simulink model "sampleModel1409"  (R2023a)
settings: Solver=VariableStepAuto  StartTime=0.0  StopTime=10.0  RelTol=1e-3
libraries: hdlsllib x3, simulink x1
settings Model: Creator=user1  LastModifiedBy=user1

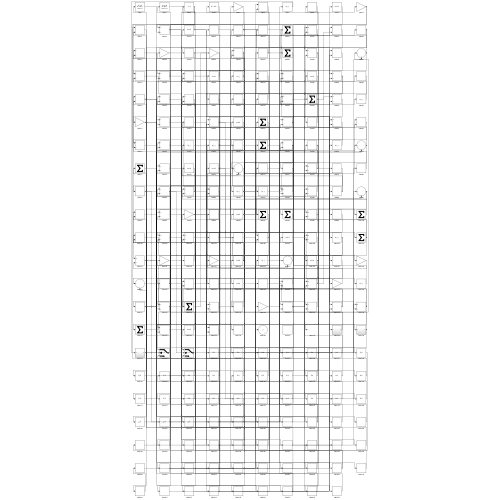
[thumbnail: Simulink's stored preview of the top-level diagram]
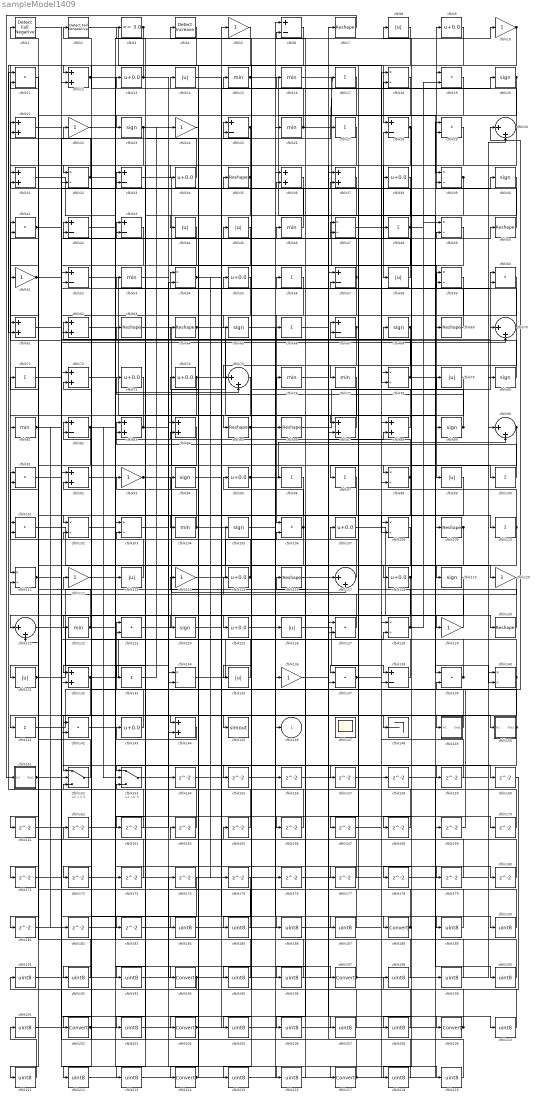
== system sampleModel1409 ==
  cfblk1 : hdlsllib/Logic and Bit Operations/Detect Fall Negative  vinit=0  OutDataTypeStr=boolean
  cfblk{5,10,22,24,51,93,112,114,120,129,136} (11 alike) : Gain
  cfblk{17,27,48,56,66,71,96..97,100,110,133,141} (12 alike) : Sum  Inputs=+
  cfblk{11,19,29,41,60,91,101,106,123,127,137,139,142} (13 alike) : DotProduct  OutDataTypeStr=Inherit: Inherit via internal rule
  cfblk{18,32,39,47,49,54,59,78,98,102..103,108,111,128,134,140} (16 alike) : Product  Inputs=*/  RndMeth=Zero  SaturateOnIntegerOverflow=on
  cfblk{15..16,26,46,53,76..77,81,104,122} (10 alike) : MinMax
  cfblk{20,23,40,65,68,80,89,94,105,119,124} (11 alike) : Signum
  cfblk{9,13,34,38,55,73..74,95,107,115,118,125,143} (13 alike) : Bias  Bias=0.0  SaturateOnIntegerOverflow=off
  cfblk{7,35,50,63..64,69,85..86,109,116,130} (11 alike) : Reshape
  cfblk{8,14,44..45,58,79,99,113,126,131,135} (11 alike) : Abs  SaturateOnIntegerOverflow=off
  cfblk{30,70,75,90,117,121} (6 alike) : Sum  Inputs=|++
  cfblk{12,21,31,36..37,61..62,72,83..84,87..88,92,132,144} (15 alike) : Sum
  cfblk{6,25,28,33,42..43,52,57,67,82,138} (11 alike) : Sum  Inputs=+-
  cfblk145 : ToWorkspace  VariableName=simout  SaveFormat=Timeseries  SampleTime=-1
  cfblk147 : Scope
      settings: Floating=on
  cfblk148 : Terminator
  cfblk149 : Subsystem
      settings: LibrarySourceBlock=|
      | hdlsllib/Ports &
      | Subsystems/Subsystem
  cfblk150 : Subsystem
      settings: LibrarySourceBlock=|
      | hdlsllib/Ports &
      | Subsystems/Subsystem
  cfblk151 : Subsystem
      settings: LibrarySourceBlock=|
      | hdlsllib/Ports &
      | Subsystems/Subsystem
  cfblk152 : Switch  SaturateOnIntegerOverflow=off  InputSameDT=off
  cfblk153 : Switch  SaturateOnIntegerOverflow=off  InputSameDT=off
  cfblk{154..183} (30 alike) : Delay  SampleTime=1
  cfblk{184..187,189..193,195..196,198..201,203,205..208,210..213,215..216,218..219} (28 alike) : DataTypeConversion  OutDataTypeStr=uint8  SaturateOnIntegerOverflow=off  RndMeth=Floor
  cfblk{188,194,197,202,204,209,214,217} (8 alike) : DataTypeConversion  SaturateOnIntegerOverflow=off  RndMeth=Floor
  cfblk2 : hdlsllib/Logic and Bit Operations/Detect Fall Nonpositive  vinit=0  OutDataTypeStr=boolean
  cfblk3 : hdlsllib/Logic and Bit Operations/Compare To Constant  relop=<=  const=3.0  OutDataTypeStr=boolean
  cfblk4 : simulink/Logic and Bit Operations/Detect Increase  vinit=0.0  OutDataTypeStr=boolean
      settings: LibrarySourceBlock=|
      | hdlsllib/Logic and Bit
      | Operations/Detect
      | Increase
  cfblk146 : Outport  VectorParamsAs1DForOutWhenUnconnected=off
  wires:
  cfblk4/1 -> cfblk111/1
  cfblk133/1 -> cfblk24/1
  cfblk90/1 -> cfblk83/2, cfblk208/1
  cfblk28/1 -> cfblk87/2, cfblk168/1
  cfblk63/1 -> cfblk98/1
  cfblk51/1 -> cfblk160/1, cfblk161/1, cfblk187/1
  cfblk141/1 -> cfblk30/1
  cfblk35/1 -> cfblk34/1, cfblk183/1
  cfblk52/1 -> cfblk85/1
  cfblk30/1 -> cfblk15/1, cfblk58/1
  cfblk83/1 -> cfblk81/1, cfblk100/1
  cfblk93/1 -> cfblk117/2, cfblk43/2, cfblk67/1
  cfblk128/1 -> cfblk62/1, cfblk19/2
  cfblk67/1 -> cfblk125/1, cfblk215/1
  cfblk16/1 -> cfblk99/1
  cfblk135/1 -> cfblk83/1
  cfblk126/1 -> cfblk138/1
  cfblk64/1 -> cfblk109/1, cfblk96/1
  cfblk14/1 -> cfblk188/1
  cfblk7/1 -> cfblk151/1(In1)
  cfblk104/1 -> cfblk33/1, cfblk120/1
  cfblk140/1 -> cfblk152/1, cfblk56/1, cfblk114/1
  cfblk113/1 -> cfblk91/1
  cfblk99/1 -> cfblk144/1
  cfblk59/1 -> cfblk106/1
  cfblk107/1 -> cfblk130/1
  cfblk132/1 -> cfblk108/1, cfblk171/1
  cfblk70/1 -> cfblk18/2, cfblk157/1
  cfblk32/1 -> cfblk21/1, cfblk108/2
  cfblk121/1 -> cfblk134/2
  cfblk10/1 -> cfblk77/1, cfblk61/2
  cfblk144/1 -> cfblk143/1
  cfblk82/1 -> cfblk121/1, cfblk153/2, cfblk49/2
  cfblk103/1 -> cfblk197/1
  cfblk120/1 -> cfblk111/2
  cfblk88/1 -> cfblk54/1
  cfblk152/1 -> cfblk71/1
  cfblk87/1 -> cfblk4/1
  cfblk109/1 -> cfblk148/1, cfblk131/1
  cfblk11/1 -> cfblk31/1
  cfblk150/1(Out1) -> cfblk42/1, cfblk193/1
  cfblk6/1 -> cfblk204/1
  cfblk36/1 -> cfblk214/1
  cfblk89/1 -> cfblk64/1, cfblk73/1
  cfblk114/1 -> cfblk106/2
  cfblk101/1 -> cfblk119/1
  cfblk58/1 -> cfblk42/2
  cfblk95/1 -> cfblk90/2, cfblk38/1
  cfblk84/1 -> cfblk152/2
  cfblk33/1 -> cfblk89/1
  cfblk26/1 -> cfblk17/1, cfblk2/1
  cfblk50/1 -> cfblk9/1
  cfblk74/1 -> cfblk136/1, cfblk142/2, cfblk175/1
  cfblk124/1 -> cfblk20/1
  cfblk18/1 -> cfblk23/1
  cfblk149/1(Out1) -> cfblk25/1
  cfblk48/1 -> cfblk13/1, cfblk102/1, cfblk49/1
  cfblk46/1 -> cfblk31/2
  cfblk80/1 -> cfblk41/1
  cfblk12/1 -> cfblk145/1, cfblk110/1
  cfblk119/1 -> cfblk141/1
  cfblk55/1 -> cfblk65/1
  cfblk138/1 -> cfblk95/1
  cfblk40/1 -> cfblk97/1
  cfblk27/1 -> cfblk61/1
  cfblk106/1 -> cfblk45/1, cfblk213/1
  cfblk131/1 -> cfblk88/2, cfblk48/1, cfblk70/2
  cfblk123/1 -> cfblk68/1
  cfblk21/1 -> cfblk129/1
  cfblk117/1 -> cfblk107/1
  cfblk75/1 -> cfblk122/1
  cfblk86/1 -> cfblk60/1
  cfblk73/1 -> cfblk142/1
  cfblk92/1 -> cfblk217/1
  cfblk98/1 -> cfblk53/1, cfblk206/1
  cfblk111/1 -> cfblk55/1, cfblk70/1
  cfblk23/1 -> cfblk212/1, cfblk216/1
  cfblk143/1 -> cfblk123/1
  cfblk56/1 -> cfblk144/2
  cfblk136/1 -> cfblk7/1
  cfblk68/1 -> cfblk135/1, cfblk178/1
  cfblk142/1 -> cfblk60/2
  cfblk76/1 -> cfblk209/1
  cfblk39/1 -> cfblk137/1, cfblk44/1
  cfblk45/1 -> cfblk124/1
  cfblk31/1 -> cfblk113/1
  cfblk72/1 -> cfblk194/1
  cfblk25/1 -> cfblk132/1, cfblk133/1
  cfblk85/1 -> cfblk57/2, cfblk170/1
  cfblk24/1 -> cfblk104/1
  cfblk139/1 -> cfblk82/1, cfblk16/1
  cfblk9/1 -> cfblk28/1
  cfblk110/1 -> cfblk118/1, cfblk67/2, cfblk47/2
  cfblk61/1 -> cfblk40/1
  cfblk47/1 -> cfblk28/2
  cfblk79/1 -> cfblk86/1
  cfblk115/1 -> cfblk63/1, cfblk102/2
  cfblk2/1 -> cfblk78/2
  cfblk153/1 -> cfblk69/1
  cfblk137/1 -> cfblk79/1, cfblk50/1
  cfblk122/1 -> cfblk11/2, cfblk166/1
  cfblk94/1 -> cfblk59/1
  cfblk62/1 -> cfblk10/1
  cfblk118/1 -> cfblk8/1, cfblk137/2
  cfblk100/1 -> cfblk35/1
  cfblk41/1 -> cfblk52/1, cfblk150/1(In1)
  cfblk97/1 -> cfblk153/1
  cfblk8/1 -> cfblk75/1
  cfblk78/1 -> cfblk46/1, cfblk140/2
  cfblk22/1 -> cfblk75/2
  cfblk69/1 -> cfblk43/1
  cfblk81/1 -> cfblk149/1(In1), cfblk182/1
  cfblk13/1 -> cfblk59/2, cfblk12/1, cfblk180/1
  cfblk116/1 -> cfblk19/1
  cfblk151/1(Out1) -> cfblk128/2, cfblk27/1
  cfblk19/1 -> cfblk51/1
  cfblk57/1 -> cfblk132/2, cfblk47/1
  cfblk127/1 -> cfblk84/2
  cfblk15/1 -> cfblk139/1, cfblk39/1
  cfblk3/1 -> cfblk32/1, cfblk12/2
  cfblk43/1 -> cfblk52/2
  cfblk134/1 -> cfblk26/1
  cfblk17/1 -> cfblk32/2
  cfblk34/1 -> cfblk3/1
  cfblk130/1 -> cfblk101/1
  cfblk20/1 -> cfblk87/1, cfblk155/1
  cfblk54/1 -> cfblk105/1, cfblk159/1
  cfblk5/1 -> cfblk202/1
  cfblk129/1 -> cfblk115/1
  cfblk53/1 -> cfblk154/1
  cfblk154/1 -> cfblk90/1
  cfblk155/1 -> cfblk138/2
  cfblk65/1 -> cfblk156/1
  cfblk157/1 -> cfblk30/2
  cfblk159/1 -> cfblk18/1
  cfblk161/1 -> cfblk54/2
  cfblk37/1 -> cfblk163/1
  cfblk163/1 -> cfblk11/1
  cfblk164/1 -> cfblk91/2
  cfblk165/1 -> cfblk121/2
  cfblk166/1 -> cfblk152/3
  cfblk60/1 -> cfblk167/1
  cfblk167/1 -> cfblk128/1
  cfblk168/1 -> cfblk134/1
  cfblk169/1 -> cfblk139/2
  cfblk170/1 -> cfblk84/1
  cfblk171/1 -> cfblk62/2
  cfblk108/1 -> cfblk172/1
  cfblk172/1 -> cfblk57/1
  cfblk42/1 -> cfblk173/1
  cfblk173/1 -> cfblk82/2
  cfblk176/1 -> cfblk98/2
  cfblk102/1 -> cfblk177/1
  cfblk177/1 -> cfblk21/2
  cfblk178/1 -> cfblk140/1
  cfblk125/1 -> cfblk179/1
  cfblk179/1 -> cfblk33/2
  cfblk180/1 -> cfblk25/2
  cfblk96/1 -> cfblk181/1
  cfblk181/1 -> cfblk78/1
  cfblk182/1 -> cfblk123/2
  cfblk183/1 -> cfblk117/1
  cfblk1/1 -> cfblk184/1
  cfblk184/1 -> cfblk126/1
  cfblk175/1 -> cfblk185/1
  cfblk185/1 -> cfblk1/1
  cfblk162/1 -> cfblk186/1
  cfblk186/1 -> cfblk127/2
  cfblk187/1 -> cfblk162/1
  cfblk188/1 -> cfblk37/2, cfblk116/1
  cfblk105/1 -> cfblk189/1
  cfblk189/1 -> cfblk14/1
  cfblk66/1 -> cfblk190/1
  cfblk190/1 -> cfblk127/1
  cfblk191/1 -> cfblk66/1
  cfblk174/1 -> cfblk192/1
  cfblk192/1 -> cfblk41/2
  cfblk193/1 -> cfblk174/1
  cfblk194/1 -> cfblk191/1, cfblk80/1
  cfblk77/1 -> cfblk195/1
  cfblk195/1 -> cfblk72/1
  cfblk156/1 -> cfblk196/1
  cfblk196/1 -> cfblk72/2
  cfblk197/1 -> cfblk39/2, cfblk22/1
  cfblk160/1 -> cfblk198/1
  cfblk198/1 -> cfblk103/1
  cfblk199/1 -> cfblk103/2
  cfblk158/1 -> cfblk200/1
  cfblk200/1 -> cfblk101/2
  cfblk201/1 -> cfblk158/1
  cfblk202/1 -> cfblk169/1, cfblk146/1
  cfblk44/1 -> cfblk203/1
  cfblk203/1 -> cfblk5/1
  cfblk204/1 -> cfblk176/1, cfblk74/1
  cfblk38/1 -> cfblk205/1
  cfblk205/1 -> cfblk6/1
  cfblk206/1 -> cfblk6/2
  cfblk112/1 -> cfblk207/1
  cfblk207/1 -> cfblk93/1
  cfblk208/1 -> cfblk112/1
  cfblk209/1 -> cfblk165/1, cfblk94/1
  cfblk91/1 -> cfblk210/1
  cfblk210/1 -> cfblk76/1
  cfblk29/1 -> cfblk211/1
  cfblk211/1 -> cfblk201/1
  cfblk212/1 -> cfblk29/1
  cfblk213/1 -> cfblk29/2
  cfblk214/1 -> cfblk164/1, cfblk88/1
  cfblk215/1 -> cfblk36/1
  cfblk216/1 -> cfblk36/2
  cfblk217/1 -> cfblk199/1, cfblk153/3, cfblk37/1
  cfblk49/1 -> cfblk218/1
  cfblk218/1 -> cfblk92/1
  cfblk71/1 -> cfblk219/1
  cfblk219/1 -> cfblk92/2

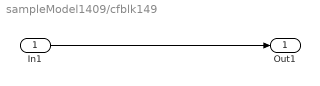
== system sampleModel1409/cfblk149 ==
  In1 : Inport
  Out1 : Outport
  wires:
  In1/1 -> Out1/1

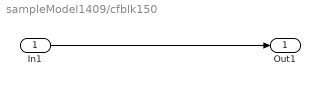
== system sampleModel1409/cfblk150 ==
  In1 : Inport
  Out1 : Outport
  wires:
  In1/1 -> Out1/1

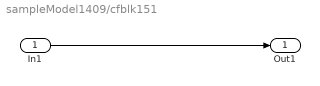
== system sampleModel1409/cfblk151 ==
  In1 : Inport
  Out1 : Outport
  wires:
  In1/1 -> Out1/1
